simulink model "VCU10"  (R2021b)
settings: Solver=FixedStepDiscrete  StartTime=0.0  StopTime=10.0  FixedStep=0.001  RelTol=1e-3
undefined symbols (not defined in the file or in its folder): F, T
libraries: simulink x146, hdlsllib x90, spsEdgeDetectorLib x2
(part 3 of 3)

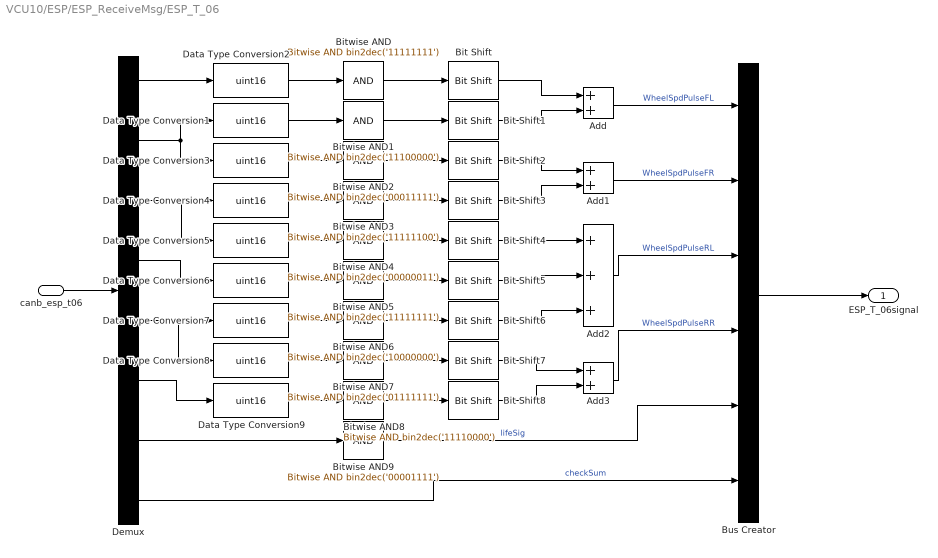
== system VCU10/ESP/ESP_ReceiveMsg/ESP_T_06 ==
  canb_esp_t06 : Inport
  Add : Sum
  Add1 : Sum
  Add2 : Sum  Inputs=+++
  Add3 : Sum
  Bit Shift : hdlsllib/Logic and Bit Operations/Bit Shift  mode=Shift Left Logical  N=3
  Bit Shift1 : hdlsllib/Logic and Bit Operations/Bit Shift  mode=Shift Right Logical  N=5
  Bit Shift2 : hdlsllib/Logic and Bit Operations/Bit Shift  mode=Shift Left Logical  N=6
  Bit Shift3 : hdlsllib/Logic and Bit Operations/Bit Shift  mode=Shift Right Logical  N=2
  Bit Shift4 : hdlsllib/Logic and Bit Operations/Bit Shift  mode=Shift Left Logical  N=9
  Bit Shift5 : hdlsllib/Logic and Bit Operations/Bit Shift  mode=Shift Left Logical  N=1
  Bit Shift6 : hdlsllib/Logic and Bit Operations/Bit Shift  mode=Shift Right Logical  N=7
  Bit Shift7 : hdlsllib/Logic and Bit Operations/Bit Shift  mode=Shift Left Logical  N=4
  Bit Shift8 : hdlsllib/Logic and Bit Operations/Bit Shift  mode=Shift Right Logical  N=4
  Bitwise AND : simulink/Logic and Bit Operations/Bitwise Operator  logicop=AND  UseBitMask=on  BitMask=bin2dec('11111111')  BitMaskRealWorld=Stored Integer
  Bitwise AND1 : simulink/Logic and Bit Operations/Bitwise Operator  logicop=AND  UseBitMask=on  BitMask=bin2dec('11100000')  BitMaskRealWorld=Stored Integer
  Bitwise AND2 : simulink/Logic and Bit Operations/Bitwise Operator  logicop=AND  UseBitMask=on  BitMask=bin2dec('00011111')  BitMaskRealWorld=Stored Integer
  Bitwise AND3 : simulink/Logic and Bit Operations/Bitwise Operator  logicop=AND  UseBitMask=on  BitMask=bin2dec('11111100')  BitMaskRealWorld=Stored Integer
  Bitwise AND4 : simulink/Logic and Bit Operations/Bitwise Operator  logicop=AND  UseBitMask=on  BitMask=bin2dec('00000011')  BitMaskRealWorld=Stored Integer
  Bitwise AND5 : simulink/Logic and Bit Operations/Bitwise Operator  logicop=AND  UseBitMask=on  BitMask=bin2dec('11111111')  BitMaskRealWorld=Stored Integer
  Bitwise AND6 : simulink/Logic and Bit Operations/Bitwise Operator  logicop=AND  UseBitMask=on  BitMask=bin2dec('10000000')  BitMaskRealWorld=Stored Integer
  Bitwise AND7 : simulink/Logic and Bit Operations/Bitwise Operator  logicop=AND  UseBitMask=on  BitMask=bin2dec('01111111')  BitMaskRealWorld=Stored Integer
  Bitwise AND8 : simulink/Logic and Bit Operations/Bitwise Operator  logicop=AND  UseBitMask=on  BitMask=bin2dec('11110000')  BitMaskRealWorld=Stored Integer
  Bitwise AND9 : simulink/Logic and Bit Operations/Bitwise Operator  logicop=AND  UseBitMask=on  BitMask=bin2dec('00001111')  BitMaskRealWorld=Stored Integer
  Bus Creator : BusCreator  Inputs=6
  Data Type Conversion{1..9} (9 alike) : DataTypeConversion  OutDataTypeStr=uint16
  Demux : Demux  Outputs=8
  ESP_T_06signal : Outport
  wires:
  canb_esp_t06/1 -> Demux/1
  Demux/1 -> Data Type Conversion2/1
  Data Type Conversion2/1 -> Bitwise AND/1
  Bitwise AND/1 -> Bit Shift/1
  Data Type Conversion1/1 -> Bitwise AND1/1
  Bitwise AND1/1 -> Bit Shift1/1
  Add/1 -> Bus Creator/1  "WheelSpdPulseFL"
  Bus Creator/1 -> ESP_T_06signal/1
  Demux/2 -> Data Type Conversion3/1, Data Type Conversion1/1
  Data Type Conversion3/1 -> Bitwise AND2/1
  Bitwise AND2/1 -> Bit Shift2/1
  Demux/3 -> Data Type Conversion5/1, Data Type Conversion4/1
  Data Type Conversion4/1 -> Bitwise AND3/1
  Bitwise AND3/1 -> Bit Shift3/1
  Add1/1 -> Bus Creator/2  "WheelSpdPulseFR"
  Bit Shift2/1 -> Add1/1
  Bit Shift3/1 -> Add1/2
  Bit Shift/1 -> Add/1
  Bit Shift1/1 -> Add/2
  Data Type Conversion5/1 -> Bitwise AND4/1
  Bitwise AND4/1 -> Bit Shift4/1
  Demux/4 -> Data Type Conversion6/1
  Data Type Conversion6/1 -> Bitwise AND5/1
  Bitwise AND5/1 -> Bit Shift5/1
  Data Type Conversion7/1 -> Bitwise AND6/1
  Bitwise AND6/1 -> Bit Shift6/1
  Bit Shift4/1 -> Add2/1
  Bit Shift5/1 -> Add2/2
  Bit Shift6/1 -> Add2/3
  Add2/1 -> Bus Creator/3  "WheelSpdPulseRL"
  Demux/5 -> Data Type Conversion8/1, Data Type Conversion7/1
  Data Type Conversion8/1 -> Bitwise AND7/1
  Bitwise AND7/1 -> Bit Shift7/1
  Demux/6 -> Data Type Conversion9/1
  Data Type Conversion9/1 -> Bitwise AND8/1
  Bitwise AND8/1 -> Bit Shift8/1
  Bit Shift7/1 -> Add3/1
  Bit Shift8/1 -> Add3/2
  Add3/1 -> Bus Creator/4  "WheelSpdPulseRR"
  Demux/7 -> Bitwise AND9/1
  Demux/8 -> Bus Creator/6  "checkSum"
  Bitwise AND9/1 -> Bus Creator/5  "lifeSig"

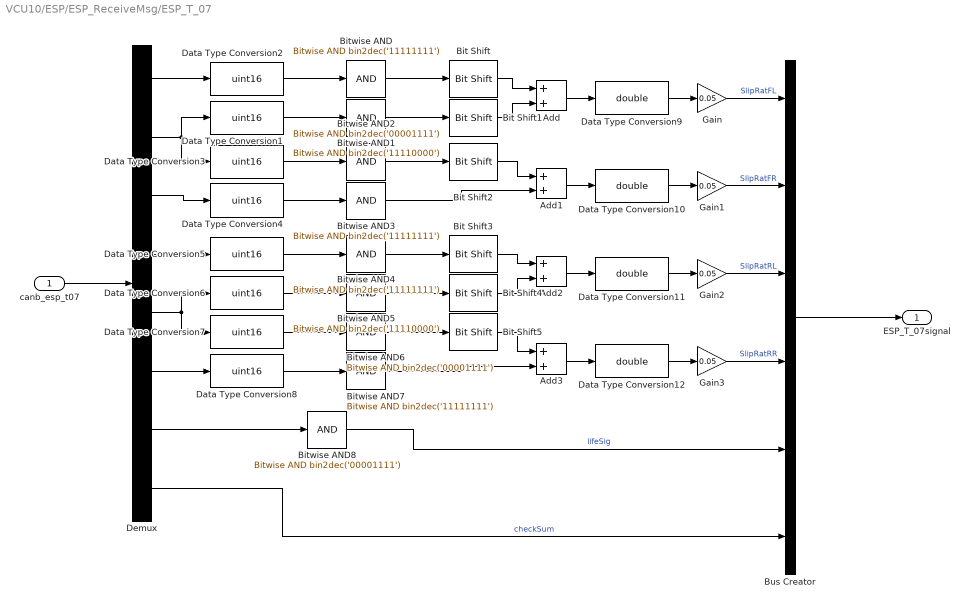
== system VCU10/ESP/ESP_ReceiveMsg/ESP_T_07 ==
  canb_esp_t07 : Inport
  Add{,1..3} (4 alike) : Sum
  Bit Shift : hdlsllib/Logic and Bit Operations/Bit Shift  mode=Shift Left Logical  N=4
  Bit Shift1 : hdlsllib/Logic and Bit Operations/Bit Shift  mode=Shift Right Logical  N=4
  Bit Shift2 : hdlsllib/Logic and Bit Operations/Bit Shift  mode=Shift Left Logical  N=8
  Bit Shift3 : hdlsllib/Logic and Bit Operations/Bit Shift  mode=Shift Left Logical  N=4
  Bit Shift4 : hdlsllib/Logic and Bit Operations/Bit Shift  mode=Shift Right Logical  N=4
  Bit Shift5 : hdlsllib/Logic and Bit Operations/Bit Shift  mode=Shift Left Logical  N=8
  Bitwise AND{,3..4,7} (4 alike) : simulink/Logic and Bit Operations/Bitwise Operator  logicop=AND  UseBitMask=on  BitMask=bin2dec('11111111')  BitMaskRealWorld=Stored Integer
  Bitwise AND1 : simulink/Logic and Bit Operations/Bitwise Operator  logicop=AND  UseBitMask=on  BitMask=bin2dec('11110000')  BitMaskRealWorld=Stored Integer
  Bitwise AND2 : simulink/Logic and Bit Operations/Bitwise Operator  logicop=AND  UseBitMask=on  BitMask=bin2dec('00001111')  BitMaskRealWorld=Stored Integer
  Bitwise AND5 : simulink/Logic and Bit Operations/Bitwise Operator  logicop=AND  UseBitMask=on  BitMask=bin2dec('11110000')  BitMaskRealWorld=Stored Integer
  Bitwise AND6 : simulink/Logic and Bit Operations/Bitwise Operator  logicop=AND  UseBitMask=on  BitMask=bin2dec('00001111')  BitMaskRealWorld=Stored Integer
  Bitwise AND8 : simulink/Logic and Bit Operations/Bitwise Operator  logicop=AND  UseBitMask=on  BitMask=bin2dec('00001111')  BitMaskRealWorld=Stored Integer
  Bus Creator : BusCreator  Inputs=6
  Data Type Conversion{1..8} (8 alike) : DataTypeConversion  OutDataTypeStr=uint16
  Data Type Conversion{9..12} (4 alike) : DataTypeConversion  OutDataTypeStr=double
  Demux : Demux  Outputs=8
  Gain{,1..3} (4 alike) : Gain  Gain=0.05
  ESP_T_07signal : Outport
  wires:
  canb_esp_t07/1 -> Demux/1
  Demux/1 -> Data Type Conversion2/1
  Demux/2 -> Data Type Conversion1/1, Data Type Conversion3/1
  Data Type Conversion1/1 -> Bitwise AND1/1
  Data Type Conversion2/1 -> Bitwise AND/1
  Bitwise AND/1 -> Bit Shift/1
  Bitwise AND1/1 -> Bit Shift1/1
  Bit Shift/1 -> Add/1
  Bit Shift1/1 -> Add/2
  Bus Creator/1 -> ESP_T_07signal/1
  Add/1 -> Data Type Conversion9/1
  Gain/1 -> Bus Creator/1  "SlipRatFL"
  Data Type Conversion3/1 -> Bitwise AND2/1
  Bitwise AND2/1 -> Bit Shift2/1
  Add1/1 -> Data Type Conversion10/1
  Gain1/1 -> Bus Creator/2  "SlipRatFR"
  Bit Shift2/1 -> Add1/1
  Demux/3 -> Data Type Conversion4/1
  Data Type Conversion4/1 -> Bitwise AND3/1
  Bitwise AND3/1 -> Add1/2
  Demux/4 -> Data Type Conversion5/1
  Data Type Conversion5/1 -> Bitwise AND4/1
  Bitwise AND4/1 -> Bit Shift3/1
  Add2/1 -> Data Type Conversion11/1
  Bit Shift3/1 -> Add2/1
  Demux/5 -> Data Type Conversion6/1, Data Type Conversion7/1
  Data Type Conversion6/1 -> Bitwise AND5/1
  Bitwise AND5/1 -> Bit Shift4/1
  Bit Shift4/1 -> Add2/2
  Gain2/1 -> Bus Creator/3  "SlipRatRL"
  Data Type Conversion7/1 -> Bitwise AND6/1
  Bitwise AND6/1 -> Bit Shift5/1
  Demux/6 -> Data Type Conversion8/1
  Data Type Conversion8/1 -> Bitwise AND7/1
  Add3/1 -> Data Type Conversion12/1
  Gain3/1 -> Bus Creator/4  "SlipRatRR"
  Bit Shift5/1 -> Add3/1
  Bitwise AND7/1 -> Add3/2
  Demux/7 -> Bitwise AND8/1
  Demux/8 -> Bus Creator/6  "checkSum"
  Data Type Conversion9/1 -> Gain/1
  Data Type Conversion10/1 -> Gain1/1
  Data Type Conversion11/1 -> Gain2/1
  Data Type Conversion12/1 -> Gain3/1
  Bitwise AND8/1 -> Bus Creator/5  "lifeSig"

== system VCU10/ESP/ESP_ReceiveMsg/Subsystem ==
  lifesig : Inport
  brkmotor_check_system : Stateflow chart  TreatAsAtomicUnit=on
  brkmotor_check : Outport
  wires:
  lifesig/1 -> brkmotor_check_system/1(lifesig)
  brkmotor_check_system/1(brkmotor_check) -> brkmotor_check/1

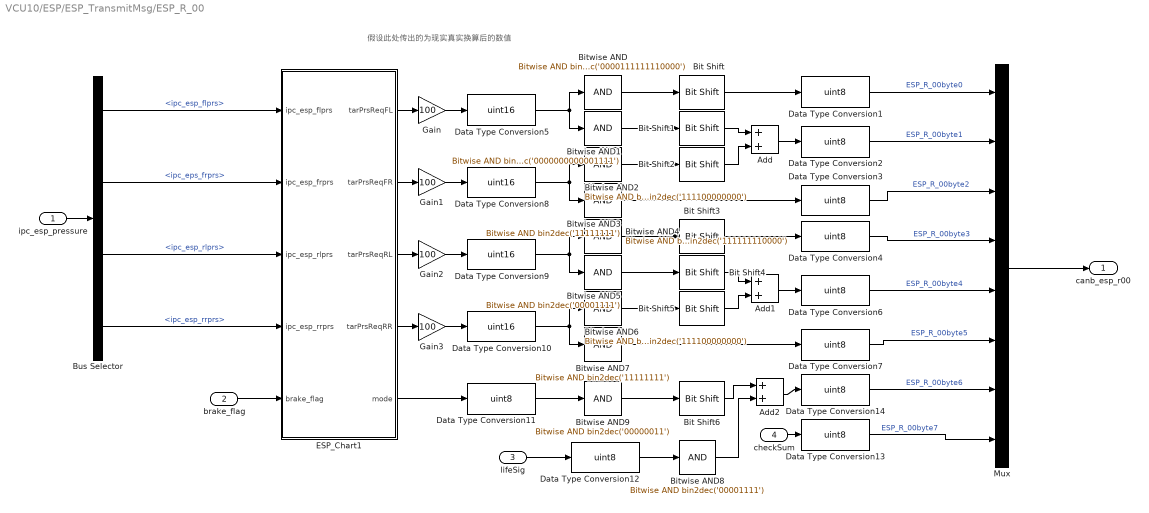
== system VCU10/ESP/ESP_TransmitMsg/ESP_R_00 ==
  note: 假设此处传出的为现实真实换算后的数值
  ipc_esp_pressure : Inport
  brake_flag : Inport  Port=2
  lifeSig : Inport  Port=3
  checkSum : Inport  Port=4
  Add : Sum
  Add1 : Sum
  Add2 : Sum
  Bit Shift : hdlsllib/Logic and Bit Operations/Bit Shift  mode=Shift Right Logical  N=4
  Bit Shift1 : hdlsllib/Logic and Bit Operations/Bit Shift  mode=Shift Left Logical  N=4
  Bit Shift2 : hdlsllib/Logic and Bit Operations/Bit Shift  mode=Shift Right Logical  N=8
  Bit Shift3 : hdlsllib/Logic and Bit Operations/Bit Shift  mode=Shift Right Logical  N=4
  Bit Shift4 : hdlsllib/Logic and Bit Operations/Bit Shift  mode=Shift Left Logical  N=4
  Bit Shift5 : hdlsllib/Logic and Bit Operations/Bit Shift  mode=Shift Right Logical  N=8
  Bit Shift6 : hdlsllib/Logic and Bit Operations/Bit Shift  mode=Shift Left Logical  N=6
  Bitwise AND : simulink/Logic and Bit Operations/Bitwise Operator  logicop=AND  UseBitMask=on  BitMask=bin2dec('0000111111110000')  BitMaskRealWorld=Stored Integer
  Bitwise AND1 : simulink/Logic and Bit Operations/Bitwise Operator  logicop=AND  UseBitMask=on  BitMask=bin2dec('0000000000001111')  BitMaskRealWorld=Stored Integer
  Bitwise AND2 : simulink/Logic and Bit Operations/Bitwise Operator  logicop=AND  UseBitMask=on  BitMask=bin2dec('111100000000')  BitMaskRealWorld=Stored Integer
  Bitwise AND3 : simulink/Logic and Bit Operations/Bitwise Operator  logicop=AND  UseBitMask=on  BitMask=bin2dec('11111111')  BitMaskRealWorld=Stored Integer
  Bitwise AND4 : simulink/Logic and Bit Operations/Bitwise Operator  logicop=AND  UseBitMask=on  BitMask=bin2dec('111111110000')  BitMaskRealWorld=Stored Integer
  Bitwise AND5 : simulink/Logic and Bit Operations/Bitwise Operator  logicop=AND  UseBitMask=on  BitMask=bin2dec('00001111')  BitMaskRealWorld=Stored Integer
  Bitwise AND6 : simulink/Logic and Bit Operations/Bitwise Operator  logicop=AND  UseBitMask=on  BitMask=bin2dec('111100000000')  BitMaskRealWorld=Stored Integer
  Bitwise AND7 : simulink/Logic and Bit Operations/Bitwise Operator  logicop=AND  UseBitMask=on  BitMask=bin2dec('11111111')  BitMaskRealWorld=Stored Integer
  Bitwise AND8 : simulink/Logic and Bit Operations/Bitwise Operator  logicop=AND  UseBitMask=on  BitMask=bin2dec('00001111')  BitMaskRealWorld=Stored Integer
  Bitwise AND9 : simulink/Logic and Bit Operations/Bitwise Operator  logicop=AND  UseBitMask=on  BitMask=bin2dec('00000011')  BitMaskRealWorld=Stored Integer
  Bus Selector : BusSelector  OutputSignals=ipc_esp_flprs,ipc_eps_frprs,ipc_esp_rlprs,ipc_esp_rrprs
  Data Type Conversion{1..4,6..7,11..14} (10 alike) : DataTypeConversion  OutDataTypeStr=uint8
  Data Type Conversion{5,8..10} (4 alike) : DataTypeConversion  OutDataTypeStr=uint16
  ESP_Chart1 : Stateflow chart  TreatAsAtomicUnit=on
  Gain{,1..3} (4 alike) : Gain  Gain=100
  Mux : Mux  Inputs=8
  canb_esp_r00 : Outport
  wires:
  Gain1/1 -> Data Type Conversion8/1
  Bitwise AND7/1 -> Data Type Conversion7/1
  Gain/1 -> Data Type Conversion5/1
  Bit Shift/1 -> Data Type Conversion1/1
  ESP_Chart1/3(tarPrsReqRL) -> Gain2/1
  Add/1 -> Data Type Conversion2/1
  Bitwise AND5/1 -> Bit Shift4/1
  Bitwise AND4/1 -> Bit Shift3/1
  Data Type Conversion1/1 -> Mux/1  "ESP_R_00byte0"
  Data Type Conversion3/1 -> Mux/3  "ESP_R_00byte2"
  brake_flag/1 -> ESP_Chart1/5(brake_flag)
  ESP_Chart1/4(tarPrsReqRR) -> Gain3/1
  Bitwise AND1/1 -> Bit Shift1/1
  Data Type Conversion4/1 -> Mux/4  "ESP_R_00byte3"
  Bit Shift2/1 -> Add/2
  Bitwise AND/1 -> Bit Shift/1
  Bitwise AND2/1 -> Bit Shift2/1
  Gain2/1 -> Data Type Conversion9/1
  Bitwise AND6/1 -> Bit Shift5/1
  Gain3/1 -> Data Type Conversion10/1
  Data Type Conversion6/1 -> Mux/5  "ESP_R_00byte4"
  Data Type Conversion2/1 -> Mux/2  "ESP_R_00byte1"
  ESP_Chart1/2(tarPrsReqFR) -> Gain1/1
  Bit Shift5/1 -> Add1/2
  Bit Shift6/1 -> Add2/1
  Bit Shift4/1 -> Add1/1
  lifeSig/1 -> Data Type Conversion12/1
  ESP_Chart1/5(mode) -> Data Type Conversion11/1
  Bit Shift3/1 -> Data Type Conversion4/1
  Bitwise AND3/1 -> Data Type Conversion3/1
  checkSum/1 -> Data Type Conversion13/1
  Add2/1 -> Data Type Conversion14/1
  Data Type Conversion7/1 -> Mux/6  "ESP_R_00byte5"
  Bitwise AND8/1 -> Add2/2
  Add1/1 -> Data Type Conversion6/1
  ESP_Chart1/1(tarPrsReqFL) -> Gain/1
  Bit Shift1/1 -> Add/1
  Data Type Conversion5/1 -> Bitwise AND1/1, Bitwise AND/1
  Data Type Conversion8/1 -> Bitwise AND3/1, Bitwise AND2/1
  Data Type Conversion9/1 -> Bitwise AND5/1, Bitwise AND4/1
  Data Type Conversion10/1 -> Bitwise AND6/1, Bitwise AND7/1
  Data Type Conversion11/1 -> Bitwise AND9/1
  Data Type Conversion12/1 -> Bitwise AND8/1
  Data Type Conversion13/1 -> Mux/8  "ESP_R_00byte7"
  Bitwise AND9/1 -> Bit Shift6/1
  ipc_esp_pressure/1 -> Bus Selector/1
  Bus Selector/1 -> ESP_Chart1/1(ipc_esp_flprs)  "<ipc_esp_flprs>"
  Bus Selector/2 -> ESP_Chart1/2(ipc_esp_frprs)  "<ipc_eps_frprs>"
  Bus Selector/3 -> ESP_Chart1/3(ipc_esp_rlprs)  "<ipc_esp_rlprs>"
  Bus Selector/4 -> ESP_Chart1/4(ipc_esp_rrprs)  "<ipc_esp_rrprs>"
  Data Type Conversion14/1 -> Mux/7  "ESP_R_00byte6"
  Mux/1 -> canb_esp_r00/1

== system VCU10/IPC/IPC_ReceiveMsg/IPC_Rx_Msg ==
  steer_return : Inport
  ipc_resgo : Inport  Port=2
  ipc_resstop : Inport  Port=3
  ipc_astask : Inport  Port=4
  Add : Sum  Inputs=+++
  Bit Shift : hdlsllib/Logic and Bit Operations/Bit Shift  mode=Shift Left Logical  N=1
  Bit Shift1 : hdlsllib/Logic and Bit Operations/Bit Shift  mode=Shift Left Logical  N=2
  Bitwise AND : simulink/Logic and Bit Operations/Bitwise Operator  logicop=AND  UseBitMask=on  BitMask=bin2dec('00000001')  BitMaskRealWorld=Stored Integer
  Bitwise AND1 : simulink/Logic and Bit Operations/Bitwise Operator  logicop=AND  UseBitMask=on  BitMask=bin2dec('00000001')  BitMaskRealWorld=Stored Integer
  Bitwise AND2 : simulink/Logic and Bit Operations/Bitwise Operator  logicop=AND  UseBitMask=on  BitMask=bin2dec('00000001')  BitMaskRealWorld=Stored Integer
  Data Type Conversion{1..4} (4 alike) : DataTypeConversion  OutDataTypeStr=uint8
  Ground : Ground
  Mux : Mux  Inputs=8
  canb_ipcrxmsg : Outport
  wires:
  Mux/1 -> canb_ipcrxmsg/1
  Ground/1 -> Mux/6, Mux/7, Mux/8, Mux/4, Mux/3, Mux/5
  Data Type Conversion1/1 -> Bitwise AND/1
  Data Type Conversion2/1 -> Bitwise AND1/1
  Bitwise AND/1 -> Add/1
  Bit Shift/1 -> Add/2
  Add/1 -> Mux/1  "canb_ipcrxmsgbyte0"
  Bitwise AND1/1 -> Bit Shift/1
  Data Type Conversion3/1 -> Mux/2  "canb_ipcrxmsgbyte1"
  Data Type Conversion4/1 -> Bitwise AND2/1
  Bitwise AND2/1 -> Bit Shift1/1
  steer_return/1 -> Data Type Conversion1/1
  ipc_resgo/1 -> Data Type Conversion2/1
  ipc_resstop/1 -> Data Type Conversion4/1
  ipc_astask/1 -> Data Type Conversion3/1
  Bit Shift1/1 -> Add/3

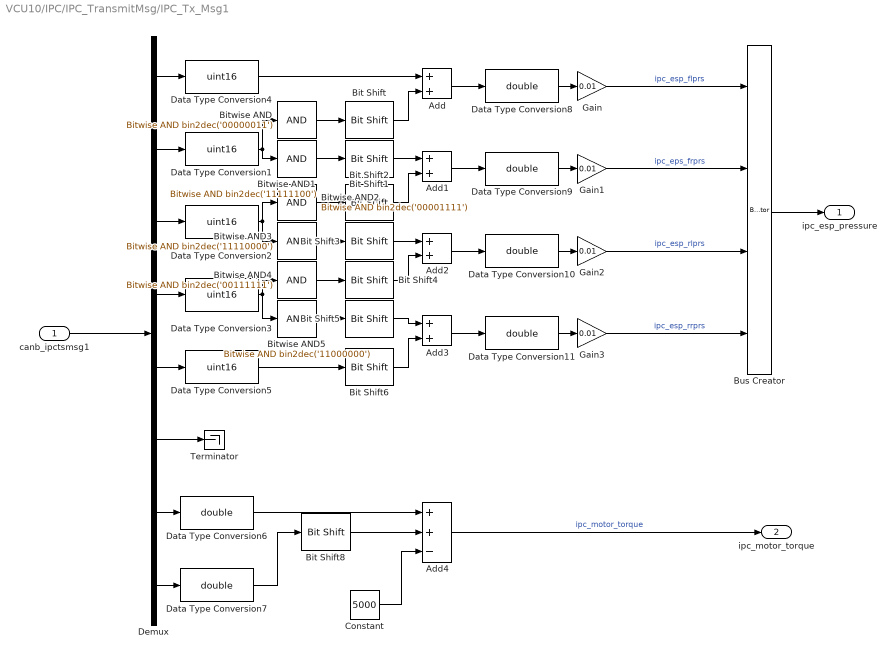
== system VCU10/IPC/IPC_TransmitMsg/IPC_Tx_Msg1 ==
  canb_ipctsmsg1 : Inport
  Add{,1..3} (4 alike) : Sum
  Add4 : Sum  Inputs=++-
  Bit Shift : hdlsllib/Logic and Bit Operations/Bit Shift  mode=Shift Left Logical  N=8
  Bit Shift1 : hdlsllib/Logic and Bit Operations/Bit Shift  mode=Shift Right Logical  N=2
  Bit Shift2 : hdlsllib/Logic and Bit Operations/Bit Shift  mode=Shift Left Logical  N=6
  Bit Shift3 : hdlsllib/Logic and Bit Operations/Bit Shift  mode=Shift Right Logical  N=4
  Bit Shift4 : hdlsllib/Logic and Bit Operations/Bit Shift  mode=Shift Left Logical  N=4
  Bit Shift5 : hdlsllib/Logic and Bit Operations/Bit Shift  mode=Shift Right Logical  N=6
  Bit Shift6 : hdlsllib/Logic and Bit Operations/Bit Shift  mode=Shift Left Logical  N=2
  Bit Shift8 : hdlsllib/Logic and Bit Operations/Bit Shift  mode=Shift Left Logical  N=8
  Bitwise AND : simulink/Logic and Bit Operations/Bitwise Operator  logicop=AND  UseBitMask=on  BitMask=bin2dec('00000011')  BitMaskRealWorld=Stored Integer
  Bitwise AND1 : simulink/Logic and Bit Operations/Bitwise Operator  logicop=AND  UseBitMask=on  BitMask=bin2dec('11111100')  BitMaskRealWorld=Stored Integer
  Bitwise AND2 : simulink/Logic and Bit Operations/Bitwise Operator  logicop=AND  UseBitMask=on  BitMask=bin2dec('00001111')  BitMaskRealWorld=Stored Integer
  Bitwise AND3 : simulink/Logic and Bit Operations/Bitwise Operator  logicop=AND  UseBitMask=on  BitMask=bin2dec('11110000')  BitMaskRealWorld=Stored Integer
  Bitwise AND4 : simulink/Logic and Bit Operations/Bitwise Operator  logicop=AND  UseBitMask=on  BitMask=bin2dec('00111111')  BitMaskRealWorld=Stored Integer
  Bitwise AND5 : simulink/Logic and Bit Operations/Bitwise Operator  logicop=AND  UseBitMask=on  BitMask=bin2dec('11000000')  BitMaskRealWorld=Stored Integer
  Bus Creator : BusCreator  Inputs=4
  Constant : Constant  Value=5000  OutDataTypeStr=uint16
  Data Type Conversion{1..5} (5 alike) : DataTypeConversion  OutDataTypeStr=uint16
  Data Type Conversion{6..11} (6 alike) : DataTypeConversion  OutDataTypeStr=double
  Demux : Demux  Outputs=8
  Gain{,1..3} (4 alike) : Gain  Gain=0.01
  Terminator : Terminator
  ipc_esp_pressure : Outport
  ipc_motor_torque : Outport  Port=2
  wires:
  canb_ipctsmsg1/1 -> Demux/1
  Demux/1 -> Data Type Conversion4/1
  Data Type Conversion1/1 -> Bitwise AND/1, Bitwise AND1/1
  Demux/2 -> Data Type Conversion1/1
  Bitwise AND/1 -> Bit Shift/1
  Data Type Conversion4/1 -> Add/1
  Bit Shift/1 -> Add/2
  Bitwise AND1/1 -> Bit Shift1/1
  Demux/3 -> Data Type Conversion2/1
  Data Type Conversion2/1 -> Bitwise AND2/1, Bitwise AND3/1
  Bitwise AND2/1 -> Bit Shift2/1
  Bit Shift1/1 -> Add1/1
  Bit Shift2/1 -> Add1/2
  Demux/4 -> Data Type Conversion3/1
  Bitwise AND3/1 -> Bit Shift3/1
  Data Type Conversion3/1 -> Bitwise AND5/1, Bitwise AND4/1
  Bitwise AND4/1 -> Bit Shift4/1
  Bit Shift4/1 -> Add2/2
  Bit Shift3/1 -> Add2/1
  Bitwise AND5/1 -> Bit Shift5/1
  Demux/5 -> Data Type Conversion5/1
  Data Type Conversion5/1 -> Bit Shift6/1
  Bit Shift5/1 -> Add3/1
  Bit Shift6/1 -> Add3/2
  Demux/6 -> Terminator/1
  Demux/7 -> Data Type Conversion6/1
  Demux/8 -> Data Type Conversion7/1
  Data Type Conversion7/1 -> Bit Shift8/1
  Data Type Conversion6/1 -> Add4/1
  Bit Shift8/1 -> Add4/2
  Bus Creator/1 -> ipc_esp_pressure/1
  Add4/1 -> ipc_motor_torque/1  "ipc_motor_torque"
  Constant/1 -> Add4/3
  Data Type Conversion8/1 -> Gain/1
  Gain/1 -> Bus Creator/1  "ipc_esp_flprs"
  Add/1 -> Data Type Conversion8/1
  Data Type Conversion9/1 -> Gain1/1
  Gain1/1 -> Bus Creator/2  "ipc_eps_frprs"
  Add1/1 -> Data Type Conversion9/1
  Data Type Conversion10/1 -> Gain2/1
  Gain2/1 -> Bus Creator/3  "ipc_esp_rlprs"
  Add2/1 -> Data Type Conversion10/1
  Data Type Conversion11/1 -> Gain3/1
  Gain3/1 -> Bus Creator/4  "ipc_esp_rrprs"
  Add3/1 -> Data Type Conversion11/1

== system VCU10/IPC/IPC_TransmitMsg/IPC_Tx_Msg2 ==
  canb_ipctsmsg2 : Inport
  Add : Sum  Inputs=++-
  Add1 : Sum
  Add2 : Sum
  Bit Shift : hdlsllib/Logic and Bit Operations/Bit Shift  mode=Shift Left Logical  N=8
  Bit Shift1 : hdlsllib/Logic and Bit Operations/Bit Shift  mode=Shift Right Logical  N=7
  Bit Shift2 : hdlsllib/Logic and Bit Operations/Bit Shift  mode=Shift Right Logical  N=6
  Bit Shift3 : hdlsllib/Logic and Bit Operations/Bit Shift  mode=Shift Right Logical  N=2
  Bit Shift4 : hdlsllib/Logic and Bit Operations/Bit Shift  mode=Shift Left Logical  N=8
  Bit Shift5 : hdlsllib/Logic and Bit Operations/Bit Shift  mode=Shift Left Logical  N=8
  Bitwise AND : simulink/Logic and Bit Operations/Bitwise Operator  logicop=AND  UseBitMask=on  BitMask=bin2dec('10000000')  BitMaskRealWorld=Stored Integer
  Bitwise AND1 : simulink/Logic and Bit Operations/Bitwise Operator  logicop=AND  UseBitMask=on  BitMask=bin2dec('01000000')  BitMaskRealWorld=Stored Integer
  Bitwise AND2 : simulink/Logic and Bit Operations/Bitwise Operator  logicop=AND  UseBitMask=on  BitMask=bin2dec('00111100')  BitMaskRealWorld=Stored Integer
  Constant : Constant  Value=1024  OutDataTypeStr=double
  Data Type Conversion1 : DataTypeConversion  OutDataTypeStr=double
  Data Type Conversion2 : DataTypeConversion  OutDataTypeStr=double
  Data Type Conversion3 : DataTypeConversion  OutDataTypeStr=boolean
  Data Type Conversion4 : DataTypeConversion  OutDataTypeStr=boolean
  Data Type Conversion5 : DataTypeConversion  OutDataTypeStr=uint8
  Data Type Conversion{6..9} (4 alike) : DataTypeConversion  OutDataTypeStr=uint16
  Demux : Demux  Outputs=8
  ipc_eps_angle : Outport
  ipc_eps_velocity : Outport  Port=2
  ipc_err : Outport  Port=3
  task_finish : Outport  Port=4
  ipc_heartbeat : Outport  Port=5
  ipc_lspd : Outport  Port=6
  ipc_hspd : Outport  Port=7
  wires:
  Add1/1 -> ipc_lspd/1
  Bit Shift3/1 -> Data Type Conversion5/1
  Demux/3 -> ipc_eps_velocity/1
  Bit Shift4/1 -> Add1/1
  Constant/1 -> Add/3
  Demux/8 -> Data Type Conversion9/1
  Data Type Conversion2/1 -> Bit Shift/1
  Data Type Conversion7/1 -> Add1/2
  Bitwise AND2/1 -> Bit Shift3/1
  Data Type Conversion8/1 -> Bit Shift5/1
  Data Type Conversion9/1 -> Add2/2
  Demux/1 -> Data Type Conversion2/1
  Bit Shift5/1 -> Add2/1
  Add2/1 -> ipc_hspd/1
  Bit Shift1/1 -> Data Type Conversion3/1
  Demux/5 -> Data Type Conversion6/1
  Data Type Conversion6/1 -> Bit Shift4/1
  Data Type Conversion5/1 -> ipc_heartbeat/1
  Demux/6 -> Data Type Conversion7/1
  Data Type Conversion4/1 -> task_finish/1
  Bit Shift2/1 -> Data Type Conversion4/1
  Demux/4 -> Bitwise AND2/1, Bitwise AND/1, Bitwise AND1/1
  Data Type Conversion3/1 -> ipc_err/1
  Add/1 -> ipc_eps_angle/1
  Bitwise AND/1 -> Bit Shift1/1
  Bitwise AND1/1 -> Bit Shift2/1
  canb_ipctsmsg2/1 -> Demux/1
  Demux/2 -> Data Type Conversion1/1
  Bit Shift/1 -> Add/1
  Data Type Conversion1/1 -> Add/2
  Demux/7 -> Data Type Conversion8/1

== system VCU10/LED_Control/EBS_LED/Enabled Subsystem ==
  In1 : Inport
  Enable : EnablePort
  Out1 : Outport
  wires:
  In1/1 -> Out1/1

== system VCU10/Res/Res_Msg/Subsystem ==
  note: 异或校验可靠性判断
  note: 赛车端与VCU断联
  note: 赛车端与遥控端断联
  res_communication : Inport
  res_heartbeat : Inport  Port=2
  res_xorcheck : Inport  Port=3
  xor_consequence : Inport  Port=4
  Logical Operator : Logic  Inputs=3  AllPortsSameDT=off  OutDataTypeStr=boolean
  heaartbeat_chart : Stateflow chart  TreatAsAtomicUnit=on
  xor_Check : Stateflow chart  TreatAsAtomicUnit=on
  res_check : Outport
  wires:
  res_heartbeat/1 -> heaartbeat_chart/1(res_heartbeat)
  heaartbeat_chart/1(res_hbcheck) -> Logical Operator/2
  res_communication/1 -> Logical Operator/1
  Logical Operator/1 -> res_check/1
  res_xorcheck/1 -> xor_Check/1(res_xorcheck)
  xor_consequence/1 -> xor_Check/2(xor_consequence)
  xor_Check/1(xorcheck) -> Logical Operator/3

== stateflow chart VCU10/AS_Stateflow/Chart ==
  state AS_Driving
    state R2D
      en:
      r2d_flag=1;
      as_ready_flag=0;
      as_driving_flag=1;
    state go
      ts_flag=1;
      r2d_flag=0;
      steering_flag=1;
      brake_flag=1;
      ebs_system_flag=1;
      as_led_yellow=2;
      as_led_blue=0;
      as_off_flag=0;
      as_ready_flag=0;
      as_driving_flag=1;
      as_finished_flag=0;
      as_emergency_flag=0;
      manual_driving_flag=0;
    (default) -> R2D
    R2D -> go : [steer_zero==1]
        | {steer_return=F;r2d_warning=F}
  state AS_Ready
    ts_flag=1;
    r2d_flag=0;
    steering_flag=1;
    brake_flag=2;
    ebs_system_flag=1;
    as_led_yellow=1;
    as_led_blue=0;
    as_off_flag=0;
    as_ready_flag=1;
    as_driving_flag=0;
    as_finished_flag=0;
    as_emergency_flag=0;
    manual_driving_flag=0;
  state transition
  state AS_Off
    ts_flag=0;
    r2d_flag=0;
    steering_flag=0;
    brake_flag=0;
    ebs_system_flag=0;
    as_led_yellow=0;
    as_led_blue=0;
    as_off_flag=1;
    as_ready_flag=0;
    as_driving_flag=0;
    as_finished_flag=0;
    as_emergency_flag=0;
    manual_driving_flag=0;
  state AS_Emergency
    ts_flag=0;
    r2d_flag=0;
    steering_flag=0;
    brake_flag=0;
    ebs_system_flag=2;
    as_led_yellow=0;
    as_led_blue=2;
    as_off_flag=0;
    as_ready_flag=0;
    as_driving_flag=0;
    as_finished_flag=0;
    as_emergency_flag=1;
    manual_driving_flag=0;
  state AS_Finished
    ts_flag=0;
    r2d_flag=0;
    steering_flag=0;
    brake_flag=0;
    ebs_system_flag=2;
    as_led_yellow=0;
    as_led_blue=1;
    as_off_flag=0;
    as_ready_flag=0;
    as_driving_flag=0;
    as_finished_flag=1;
    as_emergency_flag=0;
    manual_driving_flag=0;
  state Manual_Driving
    ts_flag=0;
    r2d_flag=0;
    steering_flag=0;
    brake_flag=0;
    ebs_system_flag=0;
    as_led_yellow=0;
    as_led_blue=0;
    as_off_flag=0;
    as_ready_flag=0;
    as_driving_flag=0;
    as_finished_flag=0;
    as_emergency_flag=0;
    manual_driving_flag=1;
  AS_Driving -> AS_Finished [order 2] : [car_spdzero==1&&task_finish==1]
      | {as_ebs_trig=1}
  AS_Ready -> (junction 54) [order 2] : after(5,sec)
  (junction 54) -> AS_Driving [order 2] : [res_go==1]
      | {r2d_warning=T;steer_return=T}
  (junction 54) -> AS_Emergency [order 1] : [ebs_working==1]
  (junction 53) -> AS_Ready [order 2] : [asb_check==1]
  AS_Driving -> (junction 136) [order 3] : [ami_inspection==1]
  AS_Ready -> AS_Emergency [order 1] : [ebs_working==1]
  AS_Driving -> AS_Emergency [order 1] : [ebs_working==1]
  (junction 53) -> AS_Emergency [order 1] : [ebs_working==1]
  transition -> (junction 53) [order 1] : [ts==1]
  (junction 136) -> AS_Emergency [order 1] : [ebs_working==1]
  (junction 136) -> AS_Finished [order 2] : after(27,sec){as_ebs_trig=1}
  transition -> AS_Emergency [order 2] : [ebs_working==1]
  AS_Off -> transition [order 2] : [as_task==1&&asms_button==1]{brake_flag=2}
  (default) -> AS_Off
  (junction 55) -> AS_Off : [asms_button==0&&brake_on==0]
  AS_Emergency -> (junction 55) : [ebs_warning==0]
  AS_Finished -> AS_Emergency [order 1] : [res_stop==1]
  AS_Off -> (junction 56) [order 1] : [ami_manualdriving==1]
  AS_Finished -> AS_Off [order 2] : [asms_button==0&&brake_on==0]
  Manual_Driving -> AS_Off : [ts==0]
  (junction 56) -> (junction 57) : [ebs_check==0]
  (junction 57) -> Manual_Driving : [ts==1]
  data: asms_button input; ebs_check input; ami_manualdriving input; as_task input; ts input; ebs_warning input; ebs_working input; brake_on input; asb_check input; car_spdzero input; task_finish input; res_go input; steer_zero input; res_stop input; as_ebs_trig output; r2d_warning output; as_led_blue output; as_led_yellow output; steer_return output; steering_flag output; brake_flag output; manual_driving_flag output; as_emergency_flag output; ebs_system_flag output; as_off_flag output; as_ready_flag output; as_driving_flag output; as_finished_flag output; r2d_flag output; ts_flag output; T parameter; F parameter; ami_inspection input

== stateflow chart VCU10/LED_Control/TSLED_Inspection ==
  state Inspection
    en:
    led_imderr=T;
    led_bmserr=T;
  state Normal
    en:
    led_imderr=F;
    led_bmserr=F;
  (default) -> Inspection
  Inspection -> Normal : [after(2,sec)]
  data: led_imderr output boolean; led_bmserr output boolean; T parameter; F parameter

== stateflow chart VCU10/TS_Activation/Chart ==
  state Ignition_Check
    state begin
      di8_flag=F;
    state DI8_Check_Flag
      (default) -> (junction 5)
      (junction 5) -> (junction 7) [order 1] : [di8_button==0]
      (junction 5) -> (junction 9) [order 2] : {di8_check_flag=0;}
      (junction 7) -> (junction 8) : {di8_check_flag=1;}
      (junction 8) -> (junction 9)
      (junction 9) -> (junction 10)
    state Check
      (default) -> (junction 23)
      (junction 23) -> (junction 25) [order 1] : [di8_button==1]
      (junction 23) -> (junction 29) [order 2]
      (junction 25) -> (junction 27) : {di8_flag=T;di8=T;}
      (junction 27) -> (junction 29)
      (junction 29) -> (junction 32)
    (default) -> begin
    begin -> DI8_Check_Flag
    (junction 17) -> DI8_Check_Flag [order 1] : [di8_check_flag==0]
    Check -> (junction 17)
    (junction 17) -> Check [order 2] : [di8_check_flag==1]
    DI8_Check_Flag -> (junction 17)
  state Flameout_Check
    state DI8_Offcheck_Flag
      (default) -> (junction 39)
      (junction 39) -> (junction 42) [order 1] : [di8_button==0]
      (junction 42) -> (junction 44) : {di8_offcheck_flag=1;}
      (junction 39) -> (junction 46) [order 2] : {di8_offcheck_flag}
      (junction 44) -> (junction 46)
      (junction 46) -> (junction 49)
    state Checkoff
      (default) -> (junction 63)
      (junction 63) -> (junction 61) [order 1] : [di8_button==1]
      (junction 63) -> (junction 57) [order 2]
      (junction 61) -> (junction 60) : {di8_flag=F;di8=F;}
      (junction 60) -> (junction 57)
      (junction 57) -> (junction 58)
    (default) -> DI8_Offcheck_Flag
    (junction 52) -> DI8_Offcheck_Flag [order 1] : [di8_offcheck_flag==0]
    (junction 52) -> Checkoff [order 3]
    (junction 52) -> Checkoff [order 2] : [di8_offcheck_flag==1]
    DI8_Offcheck_Flag -> (junction 52)
  (default) -> Ignition_Check
  Ignition_Check -> Flameout_Check : [di8_flag==T]
  Flameout_Check -> Ignition_Check : [di8_flag==F]
  data: di8_button input; di8 output boolean; di8_offcheck_flag local; di8_check_flag local; T parameter; F parameter; di8_flag local

== stateflow chart VCU10/Motor_Control/Motor_Torque_Stateflow ==
  state Default
    en:
    motor_torque=0;
  state AS_Driving
    en:
    motor_torque=as_torque;
  state Manual_Driving
    en:
    motor_torque=manual_torque;
  (default) -> Default
  Default -> AS_Driving [order 2] : [as_task==1]
  AS_Driving -> Default : [as_task==0]
  Default -> Manual_Driving [order 1] : [manual_driving_flag==1]
  Manual_Driving -> Default : [manual_driving_flag==0]
  data: manual_driving_flag input; as_task input; manual_torque input; as_torque input; motor_torque output

== stateflow chart VCU10/LED_Control/EBS_LED/display ==
  state begin
    spark=T;
  state end
    spark=F;
  (default) -> begin
  begin -> end : after(2,sec)
  data: spark output; T parameter; F parameter

== stateflow chart VCU10/TS_Activation/Chart1 ==
  state Ignition_Check
    state begin
      run_flag=0;
    state Run_Check_Flag
      (default) -> (junction 5)
      (junction 5) -> (junction 7) [order 1] : [run_button==0]
      (junction 5) -> (junction 9) [order 2] : {run_check_flag=0;}
      (junction 7) -> (junction 8) : {run_check_flag=1;}
      (junction 8) -> (junction 9)
      (junction 9) -> (junction 10)
    state Check
      (default) -> (junction 23)
      (junction 23) -> (junction 25) [order 1] : [run_button==1]
      (junction 23) -> (junction 29) [order 2]
      (junction 25) -> (junction 27) : {run_flag=1;run=T;}
      (junction 27) -> (junction 29)
      (junction 29) -> (junction 32)
    (default) -> begin
    begin -> Run_Check_Flag
    (junction 17) -> Run_Check_Flag [order 2] : [run_check_flag==0]
    Check -> (junction 17)
    (junction 17) -> Check [order 1] : [run_check_flag==1]
    Run_Check_Flag -> (junction 17)
  state Flameout_Check
    state Run_Offcheck_Flag
      (default) -> (junction 39)
      (junction 39) -> (junction 42) [order 1] : [run_button==0]
      (junction 42) -> (junction 44) : {run_offcheck_flag=1;}
      (junction 39) -> (junction 46) [order 2] : {run_offcheck_flag}
      (junction 44) -> (junction 46)
      (junction 46) -> (junction 49)
    state Checkoff
      (default) -> (junction 63)
      (junction 63) -> (junction 61) [order 1] : [run_button==1]
      (junction 63) -> (junction 57) [order 2]
      (junction 61) -> (junction 60) : {run_flag=0;run=F;}
      (junction 60) -> (junction 57)
      (junction 57) -> (junction 58)
    (default) -> Run_Offcheck_Flag
    (junction 52) -> Run_Offcheck_Flag [order 1] : [run_offcheck_flag==0]
    (junction 52) -> Checkoff [order 3]
    (junction 52) -> Checkoff [order 2] : [run_offcheck_flag==1]
    Run_Offcheck_Flag -> (junction 52)
  (default) -> Ignition_Check
  Ignition_Check -> Flameout_Check : [run_flag==1]
  Flameout_Check -> Ignition_Check : [run_flag==0]
  data: run_button input; run output boolean; run_check_flag local; run_offcheck_flag local; run_flag local; T parameter; F parameter

== stateflow chart VCU10/TS_Activation/Chart2 ==
  state begin
  state delay
  (default) -> begin
  begin -> (junction 5) : {ts=0}
  (junction 5) -> (junction 11) : [tsms_button==1]
  (junction 11) -> (junction 35) : [di8==1]
  (junction 35) -> (junction 36) [order 2] : [as_flag==1]
  (junction 35) -> (junction 7) [order 1] : [as_flag==0]
  (junction 7) -> delay : [run==1&&brake_on==1]{ts=1;ts_warning=T}
  (junction 36) -> delay : {ts=1}
  delay -> (junction 30) : after(2,sec)
  (junction 30) -> (junction 9) : {ts_warning=F}
  (junction 9) -> (junction 13) : [tsms_button==0||di8==0||run==0]{ts=0}
  (junction 13) -> (junction 15)
  data: ts output; di8 input; run input; tsms_button input; brake_on input; ts_warning output; T parameter; F parameter; as_flag input

== stateflow chart VCU10/Res/Res_Msg/Subsystem/heaartbeat_chart ==
  state begin
  state compare
    res_hbcheck=1;
  state same
    hbcnt = hbcnt + 1;
  state judge
    res_hbcheck=0;
  (default) -> begin
  begin -> compare : [hasChanged(res_heartbeat)]
  judge -> compare : [hasChanged(res_heartbeat)]
  same -> compare [order 2] : [hasChanged(res_heartbeat)]{hbcnt=0}
  compare -> same : [~hasChanged(res_heartbeat)]
  same -> judge [order 1] : [hbcnt>10]
  data: res_heartbeat input; res_hbcheck output; hbcnt local

== stateflow chart VCU10/Buzzer/Chart ==
  state Default
    en:
    ebs_buzzer=F;
  state Emergency
    en:
    ebs_buzzer=T;
  (default) -> Default
  Default -> Emergency : [as_emergency_flag==1]
  Emergency -> Default : [after(9,sec)]
  data: as_emergency_flag input; ebs_buzzer output; F parameter; T parameter

== stateflow chart VCU10/LED_Control/Subsystem/blue ==
  state Delay
    en:
    blue=uint16(60000);
  state Node
    en:
    blue=uint16(0);
  state Close
    en:
    blue=uint16(0);
  state On
    en:
    blue=uint16(60000);
  state Blink
    en:
    blue=uint16(30000);
  (default) -> Delay
  Delay -> Node : after(2,sec)
  Node -> Close [order 2] : [as_led_blue==0||asms_button==0]
  Node -> Blink [order 3] : [as_led_blue==2&&asms_button==1]
  Node -> On [order 1] : [as_led_blue==1&&asms_button==1]
  Close -> On [order 1] : [as_led_blue==1&&asms_button==1]
  On -> Blink [order 1] : [as_led_blue==2&&asms_button==1]
  Blink -> On [order 2] : [as_led_blue==1||asms_button==0]
  On -> Close [order 2] : [as_led_blue==0||asms_button==0]
  Close -> Blink [order 2] : [as_led_blue==2&&asms_button==1]
  Blink -> Close [order 1] : [as_led_blue==0||asms_button==0]
  data: as_led_blue input; blue output; asms_button input

== stateflow chart VCU10/LED_Control/Subsystem1/yellow ==
  state delay
    en:
    yellow=uint16(60000);
  state node
    en:
    yellow=uint16(0);
  state Close
    en:
    yellow=uint16(0);
  state On
    en:
    yellow=uint16(60000);
  state Blink
    en:
    yellow=uint16(30000);
  (default) -> delay
  delay -> node : after(2,sec)
  node -> Blink [order 3] : [as_led_yellow==2&&asms_button==1]
  node -> Close [order 2] : [as_led_yellow==0||asms_button==0]
  node -> On [order 1] : [as_led_yellow==1&&asms_button==1]
  Close -> On [order 1] : [as_led_yellow==1&&asms_button==1]
  On -> Blink [order 1] : [as_led_yellow==2&&asms_button==1]
  Blink -> On [order 2] : [as_led_yellow==1||asms_button==0]
  On -> Close [order 2] : [as_led_yellow==0||asms_button==0]
  Close -> Blink [order 2] : [as_led_yellow==2&&asms_button==1]
  Blink -> Close [order 1] : [as_led_yellow==0||asms_button==0]
  data: as_led_yellow input; yellow output; asms_button input

== stateflow chart VCU10/EPS/EPS_TransmitMsg/EPS_Stateflow1 ==
  state EPS_Unable
    en:
    eps_cmdworkmode=0x00;
    eps_cmdmiddle=0x00;
  state EPS_Enable
    en:
    eps_cmdworkmode=0x20;
    eps_cmdangle=ipc_cmdangle;
    eps_cmdmiddle=0x00;
    eps_cmdvelocity=ipc_eps_velocity;
  state EPS_Return
    eps_cmdworkmode=0x20;
    eps_cmdangle=uint32(0x04);
    eps_cmdmiddle=0x55;
    eps_cmdvelocity=0x14;
  (default) -> EPS_Unable
  EPS_Enable -> EPS_Unable [order 1] : [steering_flag==0]
  EPS_Unable -> EPS_Enable : [steering_flag==1]
  EPS_Enable -> (junction 22) [order 2] : [after(10,msec)]
  (junction 22) -> EPS_Return : [steer_return==1]
  EPS_Return -> EPS_Enable : [steer_zero==1]
  data: eps_cmdworkmode output; steering_flag input; steer_return input; ipc_cmdangle input; ipc_eps_velocity input; steer_zero input; eps_cmdangle output; eps_cmdmiddle output; eps_cmdvelocity output

== stateflow chart VCU10/ESP/ESP_TransmitMsg/ESP_R_00/ESP_Chart1 ==
  state ESC_Unable
    en:
    mode=0;
    %mode=机械模式;
  state ESC_Engage
    en:
    %开环模式;
    mode=1;
    tarPrsReqFL=ipc_esp_flprs;
    tarPrsReqFR=ipc_esp_frprs;
    tarPrsReqRL=ipc_esp_rlprs;
    tarPrsReqRR=ipc_esp_rrprs;
  state ESC_Able
    en:
    %开环模式;
    mode=1;
    tarPrsReqFL=ipc_esp_flprs;
    tarPrsReqFR=ipc_esp_frprs;
    tarPrsReqRL=ipc_esp_rlprs;
    tarPrsReqRR=ipc_esp_rrprs;
  (default) -> ESC_Unable
  ESC_Able -> ESC_Unable : [brake_flag==0]
  ESC_Unable -> ESC_Engage : [brake_flag==2]
  ESC_Engage -> ESC_Able : [brake_flag==1]
  data: ipc_esp_flprs input; ipc_esp_frprs input; ipc_esp_rlprs input; ipc_esp_rrprs input; brake_flag input; tarPrsReqFL output; tarPrsReqFR output; tarPrsReqRL output; tarPrsReqRR output; mode output

== stateflow chart VCU10/LED_Control/EBS_LED/Shutdown_Button ==
  state begin
  state same1
    shutdown_flag=T;
  state compare
    shutdown_count = shutdown_count + 1;
  state judge
    shutdown_flag=F;
  (default) -> begin
  begin -> (junction 28) : after(1,sec)
  (junction 28) -> same1 : [Shutdown_Start==Shutdown_End]
  judge -> same1 : [Shutdown_Start==Shutdown_End]
  compare -> same1 [order 2] : [Shutdown_Start==Shutdown_End]{shutdown_count=0}
  same1 -> compare : [Shutdown_Start~=Shutdown_End]
  compare -> judge [order 1] : [shutdown_count>10]
  data: Shutdown_Start input; shutdown_flag output; Shutdown_End input; shutdown_count local; F parameter; T parameter

== stateflow chart VCU10/ESP/ESP_ReceiveMsg/Subsystem/brkmotor_check_system ==
  state begin
  state compare
    brkmotor_check=T;
  state same
    lscnt = lscnt + 1;
  state judge
    brkmotor_check=F;
  (default) -> begin
  begin -> compare : [hasChanged(lifesig)]
  judge -> compare : [hasChanged(lifesig)]
  same -> compare [order 2] : [hasChanged(lifesig)]{lscnt=0}
  compare -> same : [~hasChanged(lifesig)]
  same -> judge [order 1] : [lscnt>10]
  data: lifesig input; brkmotor_check output; lscnt local; T parameter; F parameter

== stateflow chart VCU10/Res/Res_Msg/Subsystem/xor_Check ==
  state compare
    en:
    xorcheck=1;
  state Init
    en:
    err_cnt=0;
  state different
    en:
    err_cnt = err_cnt + 1;
  state judge
    en:
    xorcheck=0;
  (default) -> Init
  Init -> compare : [res_xorcheck==xor_consequence]
  judge -> compare : [res_xorcheck==xor_consequence]{err_cnt=0}
  compare -> different : [res_xorcheck~=xor_consequence]
  different -> compare [order 2] : [res_xorcheck==xor_consequence]{err_cnt=0}
  different -> judge [order 1] : [err_cnt>=10]
  data: res_xorcheck input; xor_consequence input; xorcheck output; err_cnt local

== stateflow chart VCU10/AMI_CAN/AMI_Transmitmsg/Chart ==
  state as_off
    en:
    ami_process=0x01
  state as_emergency
    en:
    ami_process=0x40
  state begin
  state munual_driving
    en:
    ami_process=0x02
  state as_finished
    en:
    ami_process=0x20
  state as_ready
    en:
    ami_process=0x04
  state as_driving
    en:
    ami_process=0x10
  state r2d
    en:
    ami_process=0x08
  begin -> as_off [order 1] : [as_off_flag==1]
  begin -> as_emergency [order 7] : [as_emergency_flag==1]
  as_emergency -> begin : [as_emergency_flag~=1]
  as_off -> begin : [as_off_flag~=1]
  (default) -> begin
  begin -> munual_driving [order 2] : [munual_driving_flag==1]
  begin -> as_finished [order 6] : [as_finished_flag==1]
  munual_driving -> begin : [munual_driving_flag~=1]
  as_finished -> begin : [as_finished_flag~=1]
  begin -> as_ready [order 3] : [as_ready_flag==1]
  as_ready -> begin : [as_ready_flag~=1]
  begin -> r2d [order 4] : [r2d_flag==1]
  r2d -> begin : [r2d_flag~=1]
  begin -> as_driving [order 5] : [as_driving_flag==1]
  as_driving -> begin : [as_driving_flag~=1]
  data: as_off_flag input; munual_driving_flag input; as_ready_flag input; r2d_flag input; as_driving_flag input; as_finished_flag input; as_emergency_flag input; ami_process output

== stateflow chart VCU10/Motor_Control/ManualTorque_Calculation/Pedal_Fault_Check ==
  (default) -> (junction 1)
  (junction 1) -> (junction 5) [order 1] : [abs(apps1-apps2)>=0.1]{fault_count = fault_count + 1}
  (junction 5) -> (junction 3) [order 2]
  (junction 1) -> (junction 3) [order 2] : {fault_count=0;pedal_error=0}
  (junction 5) -> (junction 10) [order 1] : [fault_count>=3]{pedal_error=1}
  (junction 10) -> (junction 3)
  (junction 3) -> (junction 13)
  data: apps1 input; apps2 input; pedal_error output; fault_count local
